simulink model "SVD_Ex3"  (R2025a)
settings: Solver=VariableStepAuto  StartTime=0.0  StopTime=10  RelTol=1e-3
undefined symbols (not defined in the file): S, static_input_Convolution_Stream_Ex1, Subsystem, vsva2197, xcvc1902
libraries: aieUtilities x3, aieSolver x1, vmcUtilities x1
settings Model: Creator=sdegala  LastModifiedBy=sdegala
settings ModelReferenceCC: EnableRefExpFcnMdlSchedulingChecks=on
settings RTWCC: GPUComputeCapability=3.5

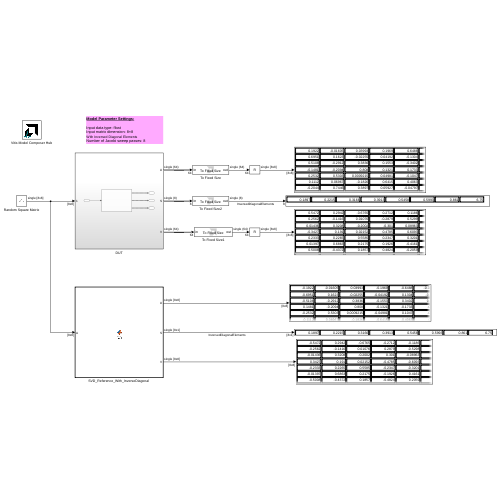
[thumbnail: Simulink's stored preview of the top-level diagram]
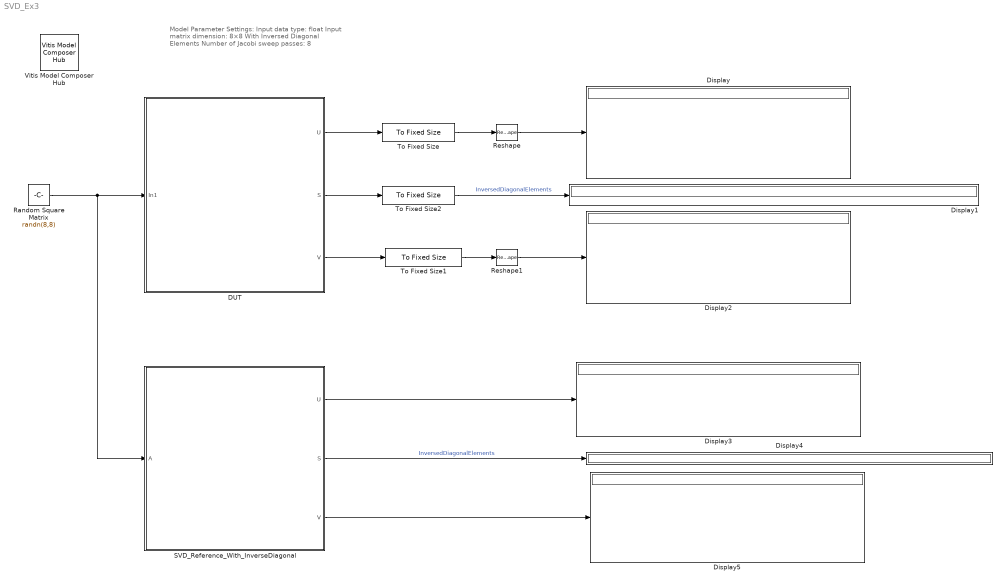
== system SVD_Ex3 ==
  note: Model Parameter Settings:
      |
      | Input data type: float
      | Input matrix dimension: 8×8
      | With Inversed Diagonal Elements
      | Number of Jacobi sweep passes: 8
  DUT : Subsystem
  Display{,1..5} (6 alike) : Display
  Random Square Matrix : Constant  Value=randn(8,8)  OutDataTypeStr=single  SampleTime=1
  Reshape : Reshape  OutputDimensionality=Customize  OutputDimensions=[8,8]
  Reshape1 : Reshape  OutputDimensionality=Customize  OutputDimensions=[8,8]
  "SVD_Reference_With_InverseDiagonal " : MATLAB Function  TreatAsAtomicUnit=on
  To Fixed Size : aieUtilities/To Fixed Size  Mode=Stop simulation when input variable-size signal is not full  OutputSize=Inherit: Same as input  CopyMethod=Buffer samples to form output  HasStatusOutput=on
  To Fixed Size1 : aieUtilities/To Fixed Size  Mode=Stop simulation when input variable-size signal is not full  OutputSize=Inherit: Same as input  CopyMethod=Buffer samples to form output  HasStatusOutput=on
  To Fixed Size2 : aieUtilities/To Fixed Size  Mode=Stop simulation when input variable-size signal is not full  OutputSize=Inherit: Same as input  CopyMethod=Buffer samples to form output  HasStatusOutput=on
  Vitis Model Composer Hub : vmcUtilities/Vitis Model Composer Hub  Tag=genX  CodeGeneration=off  SubsystemName=Subsystem  BlockHierPath=static_input_Convolution_Stream_Ex1/Subsystem  SubsystemType=AIENode  AIEArrayConfig=Use entire AIE array  StartColumn=1  NumberOfColumns=1  TargetDirectory=./code  exportDesign=on  analyzeDesign=off  validateDesignOnHw=off  ExportType=AI Engines  IpVendor=xilinx.com  IpLibrary=hls  IpVersion=1.0  IpHWLanguage=Verilog  AieCompilerOptions={}  AieSimulatorOptions={}  CreateTestbench=on  TestbenchStackSize=10  RunRtlSim=off  RunCSim=off  RunAieSim=off  enableSimulationTimeout=on  enableGraphIterations=on  AieSimTimeout=50000  AieGraphIterations=-1  RunAieSimProfiling=off  LaunchVitisAnalyzer=off  PlotOutput=off  RunX86Sim=off  X86SimTimeout=10  GenHwImage=off  GenLibadfXo=off  GenHwValidationCode=off  PlatformType=Not Specified  HwSystemType=Baremetal  HwValidationTarget=hw  ProjDevice=xcvc1902-vsva2197-1LP-e-S  ProjDevicePart=xcvc1902-vsva2197-1LP-e-S  AIEType=AIE  SamplePeriod=-1  ClockFrequency=200  DataPathParallelism=1  xilinxfamily=versalaicore  part=xcvc1902  speed=-1LP-e-S  package=vsva2197  directory=./netlist  testbench=off  incr_netlist=off  synthesis_tool=Vivado  clock_wrapper=Clock Enables  dbl_ovrd=According to Block Masks  dcm_input_clock_period=10  sysclk_period=10  simulink_period=1  eval_field=0  IPInfoJsonString="{\"DUTSubsystemName\":\"Subsystem\",\"AIESubsystem\":{\"SubsystemName\":\"Subsystem\",\"TargetDirectory\":\"./code\",\"AIEArrayConfig\":\"Use entire AIE array\",\"StartColumn\":\"0\",\"NumberOfColumns\":\"1\"},\"SubsystemTag\":\"AIENode\"}"  LogFileName=/tmp/CR-1250814/code/model_composer.log  NThreads=4  IPConfigFile=/tmp/vmctmp-13380004059271250980/static_input_Convolution_Stream_Ex1_ipconfig.json
  wires:
  To Fixed Size/1 -> Reshape/1
  To Fixed Size1/1 -> Reshape1/1
  To Fixed Size2/1 -> Display1/1  "InversedDiagonalElements"
  DUT/1(U) -> To Fixed Size/1
  DUT/2(S) -> To Fixed Size2/1
  DUT/3(V) -> To Fixed Size1/1
  Random Square Matrix/1 -> DUT/1(In1), "SVD_Reference_With_InverseDiagonal "/1(A)
  Reshape/1 -> Display/1
  Reshape1/1 -> Display2/1
  "SVD_Reference_With_InverseDiagonal "/2(S) -> Display4/1  "InversedDiagonalElements"
  "SVD_Reference_With_InverseDiagonal "/1(U) -> Display3/1
  "SVD_Reference_With_InverseDiagonal "/3(V) -> Display5/1

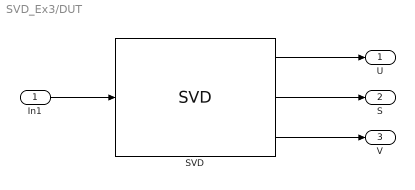
== system SVD_Ex3/DUT ==
  In1 : Inport
  SVD : aieSolver/SVD  AIE_VARIANT=1  data_type=float  row_dimension=8  cols_dimension=8  casc_length=1  num_passes=8  num_passes_ssr=1  inversion_diag=on  blockJsonConstraints=[]  blockJsonConstraintsInternal=[]  spec=vmc_svd.json  SerializedMaskParamNames=[]  SerializedMaskParamValues=[]  SerializedMaskParamVisibilities=[]  block_type=SVD  SerializedMaskParamDataypes=uint|typename|uint|uint|uint|uint|uint|uint  SerializedMaskParamEnumStrArr=0|0|0|0|0|0|0|0  SerializedMaskParamEnumValArr=0|0|0|0|0|0|0|0  SerializedMaskParamVectorArr=0|0|0|0|0|0|0|0  SerializedMaskParamKeys=AIE_VARIANT|TT_DATA|TP_DIM_ROWS|TP_DIM_COLS|TP_CASC_LEN|TP_PASSES|TP_PASSES_SSR|TP_DIAG_INV
  U : Outport
  S : Outport  Port=2
  V : Outport  Port=3
  wires:
  SVD/3 -> V/1
  SVD/1 -> U/1
  SVD/2 -> S/1
  In1/1 -> SVD/1

== matlab function SVD_Ex3/SVD_Reference_With_InverseDiagonal  ==
  data: A input; U output; S output; V output
function [U,S,V] = fcn(A)

[U,S1,V] = svd(A,"econ","vector");

S = 1./S1;
